simulink model "main_RI_LIEKF"  (R2023a)
settings: Solver=FixedStepAuto  StartTime=0.0  StopTime=220  FixedStep=0.01  RelTol=1e-3
InitFcn:
  | initNavigation0612_AOA;
values from neighbouring files (symbols this model uses):
  CF_enable = 0    [initNavigation.m]
  dt = 0.01    [initNavigation.m]
  dtDelay = -0.03    [initNavigation.m]
  g0 = 9.795    [initNavigation.m]
  gam0_rad = 0/57.3    (= 0)    [initNavigation.m]
  H_sensor_type = 0    [initNavigation.m]
  KF_enable = 1    [initNavigation.m]
  P0 = diag([1*ones(3,1);0.01*ones(3,1);0.1*ones(3,1);0.001*ones(3,1);0.00001*ones(3,1)])    [initNavigation.m]
  P0_RIEKF = diag([1*ones(3,1);0.01*ones(3,1);0.1*ones(3,1);0.001*ones(3,1);0.00001*ones(3,1);      0.01*ones(3,1);[0;2;2]/57.3;[0.1;0.1;0.1]])^2    [initNavigation.m]
  pd0 = 0    [initNavigation.m]
  pe0 = 0    [initNavigation.m]
  phi0_rad = 0/57.3    (= 0)    [initNavigation.m]
  pn0 = 0    [initNavigation.m]
  psi = -178    [initNavigation.m]
  psi0_rad = 0/57.3    (= 0)    [initNavigation.m]
  state_dim = 24    [initNavigation.m]
  Time = 0:0.01:(size(traindata.AttackAngle,1) - 1)*0.01    [NNLiftCoefficientFit.m]
  vd0 = 0    [initNavigation.m]
  ve0 = 0    [initNavigation.m]
  vn0 = 0    [initNavigation.m]
undefined symbols (not defined in the file or in its folder): DiscIntNeverNeededParam, Discrete, INS_CONST, INS_EXPORT, INS_PARAM, magnitude, p, param, pInitialization, sys
libraries: simulink x69, simulink_extras x64, dspstat3 x56, sharedtransform x49, ctrlSharedLib x36, sharedTrackingLibrary x17, FMT_Model_Lib x13, matrix_library x12, deeplib x4, dspsolvers x4, vrlib x4, aerolibconvert2 x1
(part 11 of 22)

== system main_RI_LIEKF/State estimation/RI UKF/INS propogation/att update ==
  dtheta : Inport
  gyro : Inport  Port=2
  quat_0 : Inport  Port=3  PortDimensions=4
  init_flag : Inport  Port=4
  Bus Creator1 : BusCreator  Inputs=1
  Constant : Constant  Value=dt
  Delay1 : Delay  DelayLength=1  InitialConditionSource=Input port  InitialCondition=0  ExternalReset=Level hold
      settings: InputPortMap=u0,r5,p4
  Detect Increase : simulink/Logic and Bit Operations/Detect Increase  vinit=0.0  OutDataTypeStr=boolean
  Gain1 : Gain  Commented=on  Gain=0.1
  MATLAB Function : MATLAB Function  TreatAsAtomicUnit=on
  MATLAB Function2 : MATLAB Function  TreatAsAtomicUnit=on
  Quaternions to Direction Cosine Matrix : sharedtransform/Quaternions to  Direction Cosine Matrix  aMode=aMode
      settings: LibrarySourceBlock=|
      | aerolibtransform2/Quaternions to
      | Direction Cosine Matrix
  Scope : Scope
  Transpose : Math  Operator=transpose
  att_update1 : Outport
  wires:
  init_flag/1 -> Detect Increase/1
  quat_0/1 -> Quaternions to Direction Cosine Matrix/1
  gyro/1 -> MATLAB Function/2(w)  "w"
  Constant/1 -> MATLAB Function/3(dt)
  Quaternions to Direction Cosine Matrix/1 -> Transpose/1
  Transpose/1 -> Delay1/3
  Delay1/1 -> MATLAB Function/1(Rbn_k_1)
  Detect Increase/1 -> Delay1/2
  Bus Creator1/1 -> att_update1/1
  MATLAB Function/1(Rbn) -> MATLAB Function2/2(Rbn)  "DCM_b_n"
  MATLAB Function2/1(Rbn_correct) -> Bus Creator1/1, Delay1/1  "DCM_b_n"
  dtheta/1 -> MATLAB Function2/1(delta), Scope/1

== system main_RI_LIEKF/State estimation/RI UKF/INS propogation/gyro bias compensation ==
  raw <gyro_B_rad/s_LPF> : Inport
  ddg : Inport  Port=2
  Measuemrnt Enable Flag : Inport  Port=3
  QGC_init : Inport  Port=4
  Add1 : Sum
  Data Type Conversion4 : DataTypeConversion  OutDataTypeStr=single  SaturateOnIntegerOverflow=off  RndMeth=Floor
  Scope1 : Scope
  error compensation : Subsystem
      settings: PortSchema="{\"entries\":[{\"content\":{\"sides\":[{\"content\":{\"connectorIds\":[\"In1\",\"In2\"]},\"type\":\"ConnectorPlacement.EquallySpacedRectSide\",\"uuid\":\"380e61a1-8124-48da-8c16-e78a4b6c30a9\"},{\"content\":{\"connectorIds\":[\"Out1\"],\"side\":\"RIGHT\"},\"type\":\"ConnectorPlacement.EquallySpacedRectSide\",\"uuid\":\"dacfd24e-67c3-4852-b5f7-795187362148\"},{\"content\":{\"side\":\"TOP\"},\"type\":\"ConnectorPlacement.EquallySpacedRectSide\",\"uuid\":\"56579dc4-3963-4476-a5d7-e0c30cfcd11c\"},{\"content\":{\"connectorIds\":[\"In3\"],\"side\":\"BOTTOM\"},\"type\":\"ConnectorPlacement.EquallySpacedRectSide\",\"uuid\":\"fc24e139-e918-40f2-99cc-0ca16c0a4a58\"}]},\"type\":\"ConnectorPlacement.EquallySpacedConnector\",\"uuid\":\"3ce5c04a-f8d2-476b-8ef1-0541292dfd95\"}],\"packageUris\":[\"http://schema.mathworks.com/mf0/Connector/R2020b\"],\"version\":\"1.0\"}"
  wb : Outport
  dg : Outport  Port=2
  wires:
  Data Type Conversion4/1 -> wb/1
  raw <gyro_B_rad/s_LPF>/1 -> Add1/1
  error compensation/1(dg) -> Add1/2, Scope1/1, dg/1
  Measuemrnt Enable Flag/1 -> error compensation/2(Enable)
  Add1/1 -> Data Type Conversion4/1
  QGC_init/1 -> error compensation/3(QGC_init)
  ddg/1 -> error compensation/1(ddg)

== system main_RI_LIEKF/State estimation/RI UKF/INS propogation/vel//pos update ==
  dtheta : Inport
  <DCM_b_n> : Inport  Port=2
  Ab : Inport  Port=3
  v0 : Inport  Port=4
  p0 : Inport  Port=5
  QGC_init : Inport  Port=6
  dp : Inport  Port=7
  dv : Inport  Port=8
  Kinematic Equation : Subsystem
  QGC_init1 : InportShadow  Port=6
  pos update : Subsystem
  vel update : Subsystem
  p_k : Outport
  V : Outport  Port=2
  wires:
  QGC_init1/1 -> pos update/4(QGC_init)
  pos update/1(p_k) -> p_k/1
  p0/1 -> pos update/5(p0)
  dp/1 -> pos update/3(dp)
  v0/1 -> vel update/5(v0)
  dv/1 -> vel update/4(KFState_dv)
  Kinematic Equation/1(An) -> vel update/3(An)
  QGC_init/1 -> vel update/2(QGC_init)
  Ab/1 -> Kinematic Equation/2(Ab)
  <DCM_b_n>/1 -> Kinematic Equation/1(Cbn)
  vel update/1(vel_k) -> pos update/2(vel_k), V/1
  dtheta/1 -> pos update/1(dtheta), vel update/1(dtheta)

== system main_RI_LIEKF/State estimation/bak1/Error State Kalman Filter/Cal Q1 ==
  Constant : Constant  Value=dt  OutDataTypeStr=double
  MATLAB Function1 : MATLAB Function  TreatAsAtomicUnit=on
  Qd : Outport
  wires:
  MATLAB Function1/1(Q) -> Qd/1
  Constant/1 -> MATLAB Function1/1(dt)

== system main_RI_LIEKF/State estimation/bak1/Error State Kalman Filter/Extended Kalman Filter1 ==
  Q : Inport
  Enable1 : Inport  Port=2
  y1 : Inport  Port=3
  R1 : Inport  Port=4
  BlockOrdering : Constant  Value=true()  OutDataTypeStr=boolean
  Correct1 : Subsystem  AncestorBlock=sharedTrackingLibrary/Extras/EKFCorrect  TreatAsAtomicUnit=on  SystemSampleTime=p.SampleTimes.MeasurementFcn(1)  mask(EKFCorrect){ProcessedMaskData=p}
      mask init: same as main_RI_LIEKF/State estimation/0609bk/Error State Kalman Filter/Extended Kalman Filter1/Correct1
      settings: LibrarySourceBlock=sharedTrackingLibrary/Extras/EKFCorrect
  DataStoreMemory - P : DataStoreMemory  DataStoreName=P  InitialValue=p.InitialCovariance  ShowAdditionalParam=off  OutDataTypeStr=p.DataType
  DataStoreMemory - x : DataStoreMemory  DataStoreName=x  InitialValue=p.InitialState  ShowAdditionalParam=off  OutDataTypeStr=p.DataType
  DataTypeConversion_Enable1 : DataTypeConversion  OutDataTypeStr=boolean  SaturateOnIntegerOverflow=off  RndMeth=Floor
  DataTypeConversion_Q : DataTypeConversion  OutDataTypeStr=p.DataType  SaturateOnIntegerOverflow=off  RndMeth=Floor
  DataTypeConversion_R1 : DataTypeConversion  OutDataTypeStr=p.DataType  SaturateOnIntegerOverflow=off  RndMeth=Floor
  DataTypeConversion_uMeas1 : DataTypeConversion  OutDataTypeStr=p.DataType  SaturateOnIntegerOverflow=off  RndMeth=Floor
  DataTypeConversion_uState : DataTypeConversion  OutDataTypeStr=p.DataType  SaturateOnIntegerOverflow=off  RndMeth=Floor
  DataTypeConversion_y1 : DataTypeConversion  OutDataTypeStr=p.DataType  SaturateOnIntegerOverflow=off  RndMeth=Floor
  MeasurementFcn1Inputs : Constant  Value=0  OutDataTypeStr=p.DataType  SampleTime=p.SampleTimes.MeasurementFcn(1)
  Output : Subsystem  TreatAsAtomicUnit=on  SystemSampleTime=p.SampleTimes.Output
  Predict : Subsystem  TreatAsAtomicUnit=on  SystemSampleTime=p.SampleTimes.StateTransitionFcn  mask(EKFPredict){ProcessedMaskData=p}
      mask init: same as main_RI_LIEKF/State estimation/0609bk/Error State Kalman Filter/Extended Kalman Filter1/Predict
  StateTransitionFcnInputs : Constant  Value=0  OutDataTypeStr=p.DataType  SampleTime=p.SampleTimes.StateTransitionFcn
  checkMeasurementFcn1Signals : S-Function  FunctionName=ekfukfCheckSignals  Parameters=signalCheck.BlockPath, signalCheck.MeasurementFcn{1}.PortNames, signalCheck.MeasurementFcn{1}.SampleTime, signalCheck.DataType, signalCheck.MeasurementFcn{1}.PortDimensions, 1, signalCheck.MeasurementFcn{1}.HasAdditiveNoise  SFunctionDeploymentMode=off  EnableBusSupport=off
  checkStateTransitionFcnSignals : S-Function  FunctionName=ekfukfCheckSignals  Parameters=signalCheck.BlockPath, signalCheck.StateTransitionFcn.PortNames, signalCheck.StateTransitionFcn.SampleTime, signalCheck.DataType, signalCheck.StateTransitionFcn.PortDimensions, 0, signalCheck.StateTransitionFcn.HasAdditiveNoise  SFunctionDeploymentMode=off  EnableBusSupport=off
  xhat : Outport  VectorParamsAs1DForOutWhenUnconnected=off
  P : Outport  Port=2
  wires:
  Correct1/1(yBlockOrdering) -> [AfterCorrect]
  y1/1 -> checkMeasurementFcn1Signals/2, DataTypeConversion_y1/1
  R1/1 -> checkMeasurementFcn1Signals/3, DataTypeConversion_R1/1
  Q/1 -> checkStateTransitionFcnSignals/1, DataTypeConversion_Q/1
  DataTypeConversion_Q/1 -> Predict/1(Q)
  Enable1/1 -> checkMeasurementFcn1Signals/1, DataTypeConversion_Enable1/1
  DataTypeConversion_Enable1/1 -> Correct1/Enable
  Output/2(P) -> P/1
  Output/1(x) -> xhat/1
  StateTransitionFcnInputs/1 -> checkStateTransitionFcnSignals/2, DataTypeConversion_uState/1
  DataTypeConversion_uState/1 -> Predict/2(uState)
  DataTypeConversion_y1/1 -> Correct1/1(yMeas)
  MeasurementFcn1Inputs/1 -> checkMeasurementFcn1Signals/4, DataTypeConversion_uMeas1/1
  DataTypeConversion_R1/1 -> Correct1/2(R)
  DataTypeConversion_uMeas1/1 -> Correct1/3(uMeas)
  BlockOrdering/1 -> [FirstOperation]
  [FirstOperation] -> Correct1/4(uBlockOrdering)
  [AfterCorrect] -> Output/1(uBlockOrdering)
  Output/3(yBlockOrdering) -> [AfterOutput]
  [AfterOutput] -> Predict/3(uBlockOrdering)

== system main_RI_LIEKF/State estimation/bak1/Error State Kalman Filter/Simulink Function - GPS Measurements ==
  Rbn : Inport
  vn : Inport  Port=2
  pn : Inport  Port=3
  GPSMeasurementFcn_Dyn : TriggerPort  TriggerType=function-call  IsSimulinkFunction=on  FunctionName=GPSMeasurementFcn_Dyn  VariantControl=Variant
  Add : Sum
  Data Type Conversion1 : DataTypeConversion  OutDataTypeStr=single  SaturateOnIntegerOverflow=off  RndMeth=Floor
  MATLAB Function : MATLAB Function  TreatAsAtomicUnit=on
  MATLAB Function1 : MATLAB Function  Commented=on  TreatAsAtomicUnit=on
  Product : Product  Multiplication=Matrix(*)
  pn1 : InportShadow  Port=3
  vn1 : InportShadow  Port=2
  x : ArgIn  DisableCoverage=on  OutDataTypeStr=single  PortDimensions=15  ArgumentName=x
  v : ArgIn  DisableCoverage=on  Port=2  OutDataTypeStr=single  PortDimensions=6  ArgumentName=v
  y : ArgOut  DisableCoverage=on  OutDataTypeStr=single  PortDimensions=6  ArgumentName=y
  wires:
  Data Type Conversion1/1 -> Product/1
  pn/1 -> MATLAB Function/2(pn)
  v/1 -> Add/2
  x/1 -> Product/2
  pn1/1 -> MATLAB Function1/3(pn)
  vn1/1 -> MATLAB Function1/2(vn)
  Rbn/1 -> MATLAB Function1/1(Rbn)
  vn/1 -> MATLAB Function/1(vn)
  Add/1 -> y/1
  Product/1 -> Add/1
  MATLAB Function/1(H) -> Data Type Conversion1/1

== system main_RI_LIEKF/State estimation/bak1/Error State Kalman Filter/Simulink Function - GPS Measurements1 ==
  DCM_b_n : Inport
  DynamicMeasurementFcn_Dyn : TriggerPort  TriggerType=function-call  IsSimulinkFunction=on  FunctionName=DynamicMeasurementFcn_Dyn  VariantControl=Variant
  Add : Sum  Commented=on
  Add1 : Sum
  Constant : Constant  Commented=on  Value=dt  OutDataTypeStr=single
  Constant6 : Constant  Value=[zeros(3,3),eye(3),zeros(3,12);zeros(3,15),eye(3)]  OutDataTypeStr=single
  Data Type Conversion6 : DataTypeConversion  Commented=on  OutDataTypeStr=single  SaturateOnIntegerOverflow=off  RndMeth=Floor
  From7 : From  Commented=on  GotoTag=DCM_b_n
  Goto : Goto  Commented=on  GotoTag=DCM_b_n
  MATLAB Function1 : MATLAB Function  Commented=on  TreatAsAtomicUnit=on
  Product : Product  Commented=on  Multiplication=Matrix(*)
  Product1 : Product  Multiplication=Matrix(*)
  x : ArgIn  DisableCoverage=on  OutDataTypeStr=single  PortDimensions=18  ArgumentName=x
  v : ArgIn  DisableCoverage=on  Port=2  OutDataTypeStr=single  PortDimensions=6  ArgumentName=v
  y : ArgOut  DisableCoverage=on  OutDataTypeStr=single  PortDimensions=6  ArgumentName=y
  wires:
  x/1 -> Product1/2
  Constant6/1 -> Product1/1
  Product1/1 -> Add1/1
  v/1 -> Add1/2
  Add1/1 -> y/1
  Data Type Conversion6/1 -> Product/1
  DCM_b_n/1 -> Goto/1
  Constant/1 -> MATLAB Function1/2(dt)
  From7/1 -> MATLAB Function1/1(Cbn)
  MATLAB Function1/1(H) -> Data Type Conversion6/1
  Product/1 -> Add/1

== system main_RI_LIEKF/State estimation/bak1/Error State Kalman Filter/Simulink Function - GPS Measurements2 ==
  ZUPTMeasurementFcn2 : TriggerPort  TriggerType=function-call  IsSimulinkFunction=on  FunctionName=ZUPTMeasurementFcn2  VariantControl=Variant
  Add : Sum
  Constant6 : Constant  Value=[zeros(3,3),eye(3),zeros(3,12)]  OutDataTypeStr=single
  Product : Product  Multiplication=Matrix(*)
  x : ArgIn  DisableCoverage=on  OutDataTypeStr=single  PortDimensions=18  ArgumentName=x
  v : ArgIn  DisableCoverage=on  Port=2  OutDataTypeStr=single  PortDimensions=3  ArgumentName=v
  y : ArgOut  DisableCoverage=on  OutDataTypeStr=single  PortDimensions=3  ArgumentName=y
  wires:
  v/1 -> Add/2
  Constant6/1 -> Product/1
  x/1 -> Product/2
  Product/1 -> Add/1
  Add/1 -> y/1

== system main_RI_LIEKF/State estimation/bak1/Error State Kalman Filter/Simulink Function - State Transition ==
  DCM_b_n : Inport
  vn : Inport  Port=2  PortDimensions=[3,1]
  pn : Inport  Port=3  PortDimensions=[3,1]
  stateTransitionFcn_Dyn : TriggerPort  TriggerType=function-call  IsSimulinkFunction=on  FunctionName=stateTransitionFcn_Dyn  VariantControl=Variant
  Add : Sum
  Cal Phi : Subsystem
  Constant : Constant  Value=dt  OutDataTypeStr=single
  Data Type Conversion1 : DataTypeConversion  OutDataTypeStr=single  SaturateOnIntegerOverflow=off  RndMeth=Floor
  Data Type Conversion6 : DataTypeConversion  OutDataTypeStr=single  SaturateOnIntegerOverflow=off  RndMeth=Floor
  MATLAB Function : MATLAB Function  TreatAsAtomicUnit=on
  Product1 : Product  Multiplication=Matrix(*)
  Product2 : Product  Multiplication=Matrix(*)
  x : ArgIn  DisableCoverage=on  OutDataTypeStr=single  PortDimensions=15  ArgumentName=x
  w : ArgIn  Port=2  OutDataTypeStr=single  PortDimensions=12  ArgumentName=w
  xNext : ArgOut  DisableCoverage=on  OutDataTypeStr=single  PortDimensions=15  ArgumentName=xNext
  wires:
  pn/1 -> Cal Phi/3(pn), MATLAB Function/3(pn)
  vn/1 -> Cal Phi/2(vn), MATLAB Function/2(vn)
  [DCM_b_n] -> Cal Phi/1(Rbn)
  Data Type Conversion6/1 -> Add/2
  Data Type Conversion1/1 -> Add/1
  Cal Phi/1(Phi) -> Product2/1
  DCM_b_n/1 -> [DCM_b_n]
  Constant/1 -> MATLAB Function/4(dt)
  [DCM_b_n] -> MATLAB Function/1(Rbn)
  Add/1 -> xNext/1
  Product1/1 -> Data Type Conversion1/1
  w/1 -> Product1/2
  MATLAB Function/1(G) -> Product1/1
  Product2/1 -> Data Type Conversion6/1
  x/1 -> Product2/2

== system main_RI_LIEKF/State estimation/bak1/Error State Kalman Filter/Simulink Function - State Transition Jacobian ==
  DCM_b_n : Inport
  wxyz : Inport  Port=2
  fbxyz : Inport  Port=3
  stateTransitionJacobianFcn_Dyn : TriggerPort  TriggerType=function-call  IsSimulinkFunction=on  FunctionName=stateTransitionJacobianFcn_Dyn  VariantControl=Variant
  Cal Phi : Subsystem
  Constant : Constant  Value=0.01  OutDataTypeStr=single
  Data Type Conversion1 : DataTypeConversion  OutDataTypeStr=single  SaturateOnIntegerOverflow=off  RndMeth=Floor
  Data Type Conversion6 : DataTypeConversion  OutDataTypeStr=single  SaturateOnIntegerOverflow=off  RndMeth=Floor
  MATLAB Function : MATLAB Function  TreatAsAtomicUnit=on
  Terminator : Terminator
  Terminator1 : Terminator
  Transpose : Math  Operator=transpose
  x : ArgIn  DisableCoverage=on  OutDataTypeStr=single  PortDimensions=18  ArgumentName=x
  w : ArgIn  Port=2  OutDataTypeStr=single  PortDimensions=15  ArgumentName=w
  A : ArgOut  DisableCoverage=on  OutDataTypeStr=single  PortDimensions=[18 18]  ArgumentName=A
  G : ArgOut  Port=2  OutDataTypeStr=single  PortDimensions=[18 15]  ArgumentName=G
  wires:
  Data Type Conversion1/1 -> G/1
  Data Type Conversion6/1 -> A/1
  Constant/1 -> MATLAB Function/3(dt)
  Transpose/1 -> MATLAB Function/1(Cnb)
  [DCM_b_n] -> Transpose/1
  [wxyz] -> MATLAB Function/2(wxyz)
  [DCM_b_n] -> Cal Phi/1(<DCM_b_n>)
  [fbxyz] -> Cal Phi/3(axyz)
  [wxyz] -> Cal Phi/2(wxyz)
  wxyz/1 -> [wxyz]
  fbxyz/1 -> [fbxyz]
  DCM_b_n/1 -> [DCM_b_n]
  Cal Phi/1(Phi) -> Data Type Conversion6/1
  w/1 -> Terminator1/1
  x/1 -> Terminator/1
  MATLAB Function/1(G) -> Data Type Conversion1/1

== system main_RI_LIEKF/State estimation/bak1/Error State Kalman Filter/Subsystem ==
  data : Inport
  Detect Change : simulink/Logic and Bit Operations/Detect Change  vinit=0  InputProcessing=Columns as channels (frame based)  OutDataTypeStr=boolean
  Selector : Selector  InputPortWidth=3  IndexOptions=Index vector (dialog)  Indices=[3]  OutputSizes=1
  Zero-Order Hold : ZeroOrderHold  SampleTime=0.2
  Zero-Order Hold1 : ZeroOrderHold  SampleTime=0.01
  flag : Outport
  wires:
  Zero-Order Hold/1 -> Selector/1
  data/1 -> Zero-Order Hold/1
  Selector/1 -> Zero-Order Hold1/1
  Detect Change/1 -> flag/1
  Zero-Order Hold1/1 -> Detect Change/1

== system main_RI_LIEKF/State estimation/bak1/INS propogation/Init_PVQ ==
  QGC_sensor_reinit : Inport
  accl_B_m/s2_LPF : Inport  Port=2
  Magn_B_guess_LPF : Inport  Port=3
  pos_NED : Inport  Port=4
  vel_NED : Inport  Port=5
  Constant : Constant  Value=[1 0 0 0]  OutDataTypeStr=single
  Constant1 : Constant  OutDataTypeStr=uint8
  Constant2 : Constant  Value=[0;0;0]  OutDataTypeStr=single
  Constant3 : Constant  Value=[0;0;0]  OutDataTypeStr=single
  Detect Increase : simulink/Logic and Bit Operations/Detect Increase  vinit=0.0  OutDataTypeStr=boolean
  Horizontal_attitude : Subsystem  TreatAsAtomicUnit=on
  Memory : Memory
  Scope : Scope  NumInputPorts=2
  Scope1 : Scope
  Scope2 : Scope
  Subsystem : Subsystem
  Subsystem1 : Subsystem
  Switch{,1..3} (4 alike) : Switch  Criteria=u2 > Threshold  SaturateOnIntegerOverflow=off  InputSameDT=off
  quat_0 : Outport
  v0 : Outport  Port=2
  p0 : Outport  Port=3
  wires:
  Subsystem1/1(mean_data) -> Horizontal_attitude/2(Magn_mean_B_guess_LPF)
  Subsystem/1(mean_data) -> Horizontal_attitude/1(accl_mean_B_m/s_LPF)
  Memory/1 -> Switch1/3
  Switch/1 -> quat_0/1, Scope2/1
  Horizontal_attitude/1(quat_0) -> Switch/1
  Constant/1 -> Switch/3
  Constant1/1 -> Switch1/1
  Switch1/1 -> Memory/1, Switch2/2, Switch3/2, Switch/2, Scope1/1
  accl_B_m/s2_LPF/1 -> Subsystem/1(data)
  QGC_sensor_reinit/1 -> Detect Increase/1, Scope/1
  Magn_B_guess_LPF/1 -> Subsystem1/1(data)
  Detect Increase/1 -> Horizontal_attitude/Enable, Switch1/2, Scope/2
  Constant2/1 -> Switch2/3
  Constant3/1 -> Switch3/3
  Switch2/1 -> v0/1
  Switch3/1 -> p0/1
  pos_NED/1 -> Switch3/1
  vel_NED/1 -> Switch2/1

== system main_RI_LIEKF/State estimation/bak1/INS propogation/accl bias compensation ==
  raw <accl_B_m/s2_LPF> : Inport
  dda : Inport  Port=2
  Add2 : Sum
  Data Type Conversion6 : DataTypeConversion  OutDataTypeStr=single  SaturateOnIntegerOverflow=off  RndMeth=Floor
  error compensation1 : Subsystem
  fb : Outport
  da : Outport  Port=2
  wires:
  error compensation1/1(da) -> Add2/2, da/1
  Add2/1 -> Data Type Conversion6/1
  Data Type Conversion6/1 -> fb/1
  raw <accl_B_m/s2_LPF>/1 -> Add2/1
  dda/1 -> error compensation1/1(dda)

== system main_RI_LIEKF/State estimation/bak1/INS propogation/att_update ==
  dtheta : Inport
  gyro : Inport  Port=2
  quat_0 : Inport  Port=3  PortDimensions=4
  init_flag : Inport  Port=4
  Bus Creator1 : BusCreator  Inputs=1
  Constant : Constant  Value=dt
  Delay1 : Delay  DelayLength=1  InitialConditionSource=Input port  InitialCondition=0  ExternalReset=Level hold
      settings: InputPortMap=u0,r5,p4
  Detect Increase : simulink/Logic and Bit Operations/Detect Increase  vinit=0.0  OutDataTypeStr=boolean
  MATLAB Function : MATLAB Function  TreatAsAtomicUnit=on
  MATLAB Function2 : MATLAB Function  TreatAsAtomicUnit=on
  Quaternions to Direction Cosine Matrix : sharedtransform/Quaternions to  Direction Cosine Matrix  aMode=aMode
      settings: LibrarySourceBlock=|
      | aerolibtransform2/Quaternions to
      | Direction Cosine Matrix
  Scope : Scope
  Transpose : Math  Operator=transpose
  att_update1 : Outport
  wires:
  dtheta/1 -> MATLAB Function2/1(delta), Scope/1
  MATLAB Function2/1(Rbn_correct) -> Delay1/1, Bus Creator1/1  "DCM_b_n"
  MATLAB Function/1(Rbn) -> MATLAB Function2/2(Rbn)  "DCM_b_n"
  Bus Creator1/1 -> att_update1/1
  Detect Increase/1 -> Delay1/2
  Delay1/1 -> MATLAB Function/1(Rbn_k_1)
  Transpose/1 -> Delay1/3
  Quaternions to Direction Cosine Matrix/1 -> Transpose/1
  Constant/1 -> MATLAB Function/3(dt)
  gyro/1 -> MATLAB Function/2(w)  "w"
  quat_0/1 -> Quaternions to Direction Cosine Matrix/1
  init_flag/1 -> Detect Increase/1

== system main_RI_LIEKF/State estimation/bak1/INS propogation/gyro bias compensation ==
  raw <gyro_B_rad/s_LPF> : Inport
  ddg : Inport  Port=2
  Measuemrnt Enable Flag : Inport  Port=3
  Add1 : Sum
  Data Type Conversion4 : DataTypeConversion  OutDataTypeStr=single  SaturateOnIntegerOverflow=off  RndMeth=Floor
  Scope1 : Scope
  error compensation : Subsystem
  wb : Outport
  dg : Outport  Port=2
  wires:
  ddg/1 -> error compensation/1(ddg)
  Add1/1 -> Data Type Conversion4/1
  Measuemrnt Enable Flag/1 -> error compensation/2(Enable)
  error compensation/1(dg) -> dg/1, Scope1/1, Add1/2
  raw <gyro_B_rad/s_LPF>/1 -> Add1/1
  Data Type Conversion4/1 -> wb/1

== system main_RI_LIEKF/State estimation/bak1/INS propogation/vel_pos_update ==
  dtheta : Inport
  <DCM_b_n> : Inport  Port=2
  Ab : Inport  Port=3
  v0 : Inport  Port=4
  p0 : Inport  Port=5
  QGC_init : Inport  Port=6
  dp : Inport  Port=7
  dv : Inport  Port=8
  Kinematic Equation : Subsystem
  QGC_init1 : InportShadow  Port=6
  pos update : Subsystem
  vel update : Subsystem
  p_k : Outport
  V : Outport  Port=2
  wires:
  dtheta/1 -> vel update/1(dtheta), pos update/1(dtheta)
  vel update/1(vel_k) -> V/1, pos update/2(vel_k)
  <DCM_b_n>/1 -> Kinematic Equation/1(Cbn)
  Ab/1 -> Kinematic Equation/2(Ab)
  QGC_init/1 -> vel update/2(QGC_init)
  Kinematic Equation/1(An) -> vel update/3(An)
  dv/1 -> vel update/4(KFState_dv)
  v0/1 -> vel update/5(v0)
  dp/1 -> pos update/3(dp)
  p0/1 -> pos update/5(p0)
  pos update/1(p_k) -> p_k/1
  QGC_init1/1 -> pos update/4(QGC_init)

== system main_RI_LIEKF/State estimation/distribute CF/AHRS/AHRS Complementary filter ==
  fbxyz : Inport
  Q_update : Inport  Port=2
  GPS_Data : Inport  Port=3
  magxyz : Inport  Port=4
  reset : Inport  Port=5
  Bus Selector : BusSelector  OutputSignals=vn_gps,ve_gps,vd_gps
  Bus Selector1 : BusSelector  OutputSignals=DCM_b_n
  Bus Selector2 : BusSelector  OutputSignals=fixtype_gps
  Compare To Constant : simulink/Logic and Bit Operations/Compare To Constant  relop=<=  const=2  OutDataTypeStr=boolean
  Complementary Filter : Subsystem
  Constant : Constant  Value=zeros(3,1)  OutDataTypeStr=single
  Discrete-Time Integrator2 : DiscreteIntegrator  Commented=on  ExternalReset=rising  SampleTime=-1  LimitOutput=on  UpperSaturationLimit=0.005  LowerSaturationLimit=-0.005  ICPrevOutput=DiscIntNeverNeededParam  ICPrevScaledInput=DiscIntNeverNeededParam
  GPSHeadingCorrect : Subsystem
  Gain1 : Gain  Gain=[1;1;0]
  Gain3 : Gain  Commented=on  Gain=0.01
  MagnHeadingCorrect : Subsystem
  Q_update1 : InportShadow  Port=2
  Scope{,2..4,6} (5 alike) : Scope
  Scope1 : Scope  NumInputPorts=2
  Scope5 : Scope  NumInputPorts=2
  Sum : Sum  Inputs=|+--
  Switch : Switch  Threshold=3  SaturateOnIntegerOverflow=off  InputSameDT=off
  Terminator1 : Terminator
  Trace differentiator : Subsystem
  UAV_accelerate_within_gravity_estimate : Subsystem
  Vector Concatenate : Concatenate  NumInputs=3
  fbxyz1 : InportShadow
  gyro_preprocessing2 : Subsystem
  manoeuvrable check : Subsystem
  w_bias : Outport
  wires:
  Switch/1 -> Gain1/1
  gyro_preprocessing2/1(gyro_B_rad/s_LPF) -> Gain3/1, w_bias/1, Scope6/1
  Complementary Filter/1(w_bias) -> Switch/3
  reset/1 -> Discrete-Time Integrator2/2
  Constant/1 -> Switch/1
  Sum/1 -> gyro_preprocessing2/1(gyro_B_rad/s_ori)
  Gain3/1 -> Discrete-Time Integrator2/1
  MagnHeadingCorrect/1(wz_bias_by_magn) -> Scope1/1, Sum/3
  magxyz/1 -> MagnHeadingCorrect/2(Magnxyz), Scope1/2
  GPSHeadingCorrect/2(PsiGPS&pitch&roll) -> Terminator1/1
  GPSHeadingCorrect/1(wz_bias_by_GPS) -> Sum/2, Scope/1
  Q_update1/1 -> GPSHeadingCorrect/2(Q_update)
  Gain1/1 -> Sum/1
  manoeuvrable check/1(Fly_status) -> Compare To Constant/1, Switch/2, Scope3/1, Complementary Filter/2(Fly_status), UAV_accelerate_within_gravity_estimate/1(Fly_status)
  Bus Selector2/1 -> manoeuvrable check/4(fixtype_GPS), UAV_accelerate_within_gravity_estimate/2(GPS_type)  "<fixtype_gps>"
  fbxyz1/1 -> manoeuvrable check/2(fbxyz1)
  Trace differentiator/1(originalVariableDifference) -> UAV_accelerate_within_gravity_estimate/4(accel_GPS_ned), manoeuvrable check/1(accel_GPS_ned), Scope5/1  "accel_GPS_ned"
  UAV_accelerate_within_gravity_estimate/1(accelerate_within_gravity_estimate) -> Scope2/1, Complementary Filter/3(fb_estimatedValue)
  fbxyz/1 -> Complementary Filter/1(fbxyz)
  Vector Concatenate/1 -> Trace differentiator/1(originalVariable), Scope5/2, Scope4/1  "v_GPS_ned"
  Bus Selector1/1 -> MagnHeadingCorrect/1(Cbn), manoeuvrable check/3(DCM_b_n), UAV_accelerate_within_gravity_estimate/3(<DCM_b_n>)  "<DCM_b_n>"
  Q_update/1 -> Bus Selector1/1
  Bus Selector/3 -> Vector Concatenate/3  "<vd_gps>"
  Bus Selector/2 -> Vector Concatenate/2  "<ve_gps>"
  Bus Selector/1 -> Vector Concatenate/1  "<vn_gps>"
  GPS_Data/1 -> Bus Selector/1, GPSHeadingCorrect/1(GPSdata), Bus Selector2/1

== system main_RI_LIEKF/State estimation/distribute CF/AHRS/Init_Q0 ==
  QGC_sensor_reinit : Inport
  accl_B_m/s2_LPF : Inport  Port=2
  Magn_B_guess_LPF : Inport  Port=3
  Constant : Constant  Value=[1 0 0 0]  OutDataTypeStr=single
  Constant1 : Constant  OutDataTypeStr=uint8
  Detect Increase : simulink/Logic and Bit Operations/Detect Increase  vinit=0.0  OutDataTypeStr=boolean
  Horizontal_attitude : Subsystem  TreatAsAtomicUnit=on
  Memory : Memory
  Scope : Scope  NumInputPorts=2
  Scope1 : Scope
  Scope2 : Scope
  Subsystem : Subsystem
  Subsystem1 : Subsystem
  Switch : Switch  Criteria=u2 > Threshold  SaturateOnIntegerOverflow=off  InputSameDT=off
  Switch1 : Switch  Criteria=u2 > Threshold  SaturateOnIntegerOverflow=off  InputSameDT=off
  quat_0 : Outport
  wires:
  Subsystem1/1(mean_data) -> Horizontal_attitude/2(Magn_mean_B_guess_LPF)
  Subsystem/1(mean_data) -> Horizontal_attitude/1(accl_mean_B_m/s_LPF)
  Memory/1 -> Switch1/3
  Switch/1 -> quat_0/1, Scope2/1
  Horizontal_attitude/1(quat_0) -> Switch/1
  Constant/1 -> Switch/3
  Constant1/1 -> Switch1/1
  Switch1/1 -> Memory/1, Switch/2, Scope1/1
  accl_B_m/s2_LPF/1 -> Subsystem/1(data)
  QGC_sensor_reinit/1 -> Detect Increase/1, Scope/1
  Magn_B_guess_LPF/1 -> Subsystem1/1(data)
  Detect Increase/1 -> Horizontal_attitude/Enable, Switch1/2, Scope/2

== system main_RI_LIEKF/State estimation/distribute CF/AHRS/att_update ==
  Sensor_data : Inport
  quat_0 : Inport  Port=2  PortDimensions=4
  init_flag : Inport  Port=3
  wbias : Inport  Port=4  PortDimensions=3
  Add : Sum
  Bus Creator : BusCreator  Inputs=2
  Bus Selector1 : BusSelector  OutputSignals=IMU_Data.gyro_B_rad/s_LPF
  Delay : Delay  DelayLength=1  InitialConditionSource=Input port  ExternalReset=Level hold
      settings: InputPortMap=u0,r5,p4
  Detect Increase : simulink/Logic and Bit Operations/Detect Increase  vinit=0.0  OutDataTypeStr=boolean
  Gain : Gain  Gain=dt
  Memory : Memory  InitialCondition=zeros(3,1)  InheritSampleTime=on
  QuatMult : MATLAB Function  TreatAsAtomicUnit=on
  Quaternions to Direction Cosine Matrix : sharedtransform/Quaternions to  Direction Cosine Matrix  aMode=aMode
  Scope : Scope
  Scope1 : Scope
  Transpose : Math  Operator=transpose  SignedPower=on
  rv2q : MATLAB Function  TreatAsAtomicUnit=on
  uniformization : Subsystem
  att_update : Outport
  wires:
  uniformization/1(Q o) -> Bus Creator/1, Delay/1, Quaternions to Direction Cosine Matrix/1  "q_update"
  Memory/1 -> Add/2
  wbias/1 -> Memory/1
  Detect Increase/1 -> Delay/2
  init_flag/1 -> Detect Increase/1
  Bus Creator/1 -> att_update/1
  Transpose/1 -> Bus Creator/2  "DCM_b_n"
  Quaternions to Direction Cosine Matrix/1 -> Transpose/1
  quat_0/1 -> Delay/3
  Delay/1 -> QuatMult/1(quatA)
  QuatMult/1(quatOut) -> uniformization/1(Q i)  "q_update"
  Sensor_data/1 -> Bus Selector1/1
  Gain/1 -> rv2q/1(rotVec)  "correctedDelAng"
  Bus Selector1/1 -> Add/1, Scope1/1  "<gyro_B_rad/s_LPF>"
  Add/1 -> Gain/1
  rv2q/1(quaternion) -> QuatMult/2(quatB)

== system main_RI_LIEKF/State estimation/distribute CF/Translation_estimate/Rxy_Horizontal_estimation ==
  Vn : Inport
  Enable : Inport  Port=2
  Sensor_data2 : Inport  Port=3
  Add1 : Sum  Inputs=+-
  Bus Selector1 : BusSelector  OutputSignals=GPS_Data.pos_N_gps,GPS_Data.pos_E_gps
  Delay1 : Delay  DelayLength=1
  Integrator_R_Horizontal : Subsystem
  Mux1 : Mux  Inputs=2
  Rxy_kalman filter2 : Subsystem  mask{F=diag([-0.1,-0.1,-0.01,-0.01]), H=[1,0,-1,0;0,1,0,-1], Q=diag([1,1,0.1,0.1]), R=diag([0.05,0.05]), P0=diag([0.8,0.8,0.2,0.2])}
      mask prompts: F "状态转移矩阵：F"; H "观测转移矩阵：H"; Q "预测噪声协方差矩阵：Q"; R "量测噪声协方差矩阵：R"; P0 "初始协方差矩阵：P0"
      mask DialogControl DescTextVar Prompt: Kalman Filter
  Scope1 : Scope  NumInputPorts=2
  Selector1 : Selector  InputPortWidth=4  IndexOptions=Index vector (dialog)  Indices=[1 2]  OutputSizes=1
  R_n&e : Outport
  wires:
  Vn/1 -> Integrator_R_Horizontal/1(Vn)
  Add1/1 -> Rxy_kalman filter2/2(Z)
  Rxy_kalman filter2/1(XOut) -> Delay1/1
  Enable/1 -> Rxy_kalman filter2/3(Enable)
  Bus Selector1/1 -> Mux1/1  "<pos_N_gps>"
  Integrator_R_Horizontal/1(R_n&e) -> Add1/1, Scope1/1, R_n&e/1
  Bus Selector1/2 -> Mux1/2  "<pos_E_gps>"
  Sensor_data2/1 -> Bus Selector1/1, Integrator_R_Horizontal/3(Sensor_data2)
  Delay1/1 -> Rxy_kalman filter2/1(X), Selector1/1
  Mux1/1 -> Scope1/2, Add1/2
  Selector1/1 -> Integrator_R_Horizontal/2(dR)

== system main_RI_LIEKF/State estimation/distribute CF/Translation_estimate/V_Horizontal_estimation ==
  note: 0530改：
      | 加入GPStype限制
  An : Inport
  Sensor_data2 : Inport  Port=2
  Add : Sum  Inputs=+-
  Bus Selector2 : BusSelector  OutputSignals=GPS_Data.vn_gps,GPS_Data.ve_gps,GPS_Data.fixtype_gps
  Compare To Constant : simulink/Logic and Bit Operations/Compare To Constant  relop=>=  const=1  OutDataTypeStr=boolean
  Delay : Delay  DelayLength=1
  Detect Change : simulink/Logic and Bit Operations/Detect Change  vinit=0  OutDataTypeStr=boolean
  Integrator_V_Horizontal : Subsystem
  Logical Operator : Logic  AllPortsSameDT=off  OutDataTypeStr=boolean
  Mux : Mux  Inputs=2
  Rxy_kalman filter1 : Subsystem  mask{F=diag([-0.1,-0.1,-0.01,-0.01]), H=[1,0,-1,0;0,1,0,-1], Q=diag([1,1,0.1,0.1]), R=diag([0.1,0.1]), P0=diag([0.8,0.8,0.5,0.5])}
      mask prompts: F "状态转移矩阵：F"; H "观测转移矩阵：H"; Q "预测噪声协方差矩阵：Q"; R "量测噪声协方差矩阵：R"; P0 "初始协方差矩阵：P0"
      mask DialogControl DescTextVar Prompt: Kalman Filter
  Scope : Scope  NumInputPorts=2
  Scope1 : Scope
  Selector : Selector  InputPortWidth=4  IndexOptions=Index vector (dialog)  Indices=[1 2]  OutputSizes=1
  vxy_estimout : Outport
  V_n&e : Outport  Port=2
  GPS_v_enable : Outport  Port=3
  wires:
  Logical Operator/1 -> Rxy_kalman filter1/3(Enable), Scope1/1, GPS_v_enable/1
  Compare To Constant/1 -> Logical Operator/2
  Detect Change/1 -> Logical Operator/1
  Bus Selector2/3 -> Compare To Constant/1  "<fixtype_gps>"
  Sensor_data2/1 -> Integrator_V_Horizontal/3(Sensor_data2), Bus Selector2/1
  An/1 -> Integrator_V_Horizontal/1(An)
  Add/1 -> Rxy_kalman filter1/2(Z)
  Integrator_V_Horizontal/1(V_n&e) -> Add/1, Scope/1, vxy_estimout/1, V_n&e/1
  Rxy_kalman filter1/1(XOut) -> Delay/1
  Bus Selector2/2 -> Mux/2  "<ve_gps>"
  Mux/1 -> Add/2, Scope/2
  Bus Selector2/1 -> Detect Change/1, Mux/1  "<vn_gps>"
  Selector/1 -> Integrator_V_Horizontal/2(dv)
  Delay/1 -> Rxy_kalman filter1/1(X), Selector/1

== system main_RI_LIEKF/State estimation/distribute CF/Translation_estimate/translate to N ==
  RotationData : Inport
  Sensor_data : Inport  Port=2
  Bus Selector2 : BusSelector  OutputSignals=IMU_Data.accl_B_m/s2_LPF
  Bus Selector3 : BusSelector  OutputSignals=DCM_b_n
  Product : Product  Multiplication=Matrix(*)
  Selector : Selector  InputPortWidth=3  IndexOptions=Index vector (dialog)  Indices=[1 2]  OutputSizes=1
  Selector1 : Selector  InputPortWidth=3  IndexOptions=Index vector (dialog)  Indices=[3]  OutputSizes=1
  accel_Horizontal_predict : Outport
  accel_Vertical_predict : Outport  Port=2
  wires:
  Selector1/1 -> accel_Vertical_predict/1
  Selector/1 -> accel_Horizontal_predict/1
  Product/1 -> Selector/1, Selector1/1
  Sensor_data/1 -> Bus Selector2/1
  Bus Selector3/1 -> Product/1  "<DCM_b_n>"
  Bus Selector2/1 -> Product/2  "<accl_B_m/s2_LPF>"
  RotationData/1 -> Bus Selector3/1

== system main_RI_LIEKF/State estimation/distribute CF/distribute CF/AHRS1 ==
  RF_Data : Inport
  Sensor_Data : Inport  Port=2
  Bus_Constructor : Subsystem  TreatAsAtomicUnit=on
  Correct : Subsystem  TreatAsAtomicUnit=on
  Delay : Delay  DelayLength=1
  Update : Subsystem  TreatAsAtomicUnit=on
  Rotation_Data : Outport
  wires:
  Correct/1(att_B_correction) -> Update/1(att_B_correction)
  Bus_Constructor/1(Rotation_Data) -> Delay/1, Rotation_Data/1
  Correct/2(bias_g_B_correction) -> Update/2(bias_g_correction)
  Sensor_Data/1 -> Bus_Constructor/5(Sensor_Data), Update/4(Sensor_Data), Correct/2(Sensor_Data)
  Update/1(att_quat) -> Bus_Constructor/2(att_quat)
  Update/2(DCM_OB) -> Bus_Constructor/3(DCM_OB)
  Update/3(bias_g) -> Bus_Constructor/4(bias_g)
  RF_Data/1 -> Correct/3(RF_Data), Bus_Constructor/1(RF_Data), Update/3(RF_Data)
  Delay/1 -> Correct/1(Rotation_Data)

== system main_RI_LIEKF/State estimation/distribute CF/distribute CF/Bus_Constructor ==
  RF_Data : Inport
  att_quat : Inport  Port=2
  DCM_OB : Inport  Port=3
  bias_g : Inport  Port=4
  gyro_B_correction : Inport  Port=5
  Sensor_Data : Inport  Port=6
  Bus Creator : BusCreator  Inputs=12
  Bus Selector : BusSelector  OutputSignals=IMU_Data.gyro_B_rad/s_LPF,IMU_Data.accl_B_m/s2_LPF
  Bus Selector1 : BusSelector  OutputSignals=att_reset
  Constant : Constant
  Euler_Angle : Subsystem
  Math Function : Math  Operator=transpose  SignedPower=on
  Signal Conversion{,1..4} (5 alike) : SignalConversion  OverrideOpt=off
  Subsystem1 : Subsystem
  Terminator2 : Terminator
  Rotation_Data : Outport
  wires:
  Bus Selector1/1 -> Signal Conversion4/1  "<att_reset>"
  Signal Conversion/1 -> Bus Creator/11  "acc_B_mPs2"
  Euler_Angle/1(phi_rad) -> Bus Creator/2  "phi_rad"
  Euler_Angle/2(theta_rad) -> Bus Creator/3  "theta_rad"
  Euler_Angle/3(psi_rad) -> Subsystem1/1(psi), Bus Creator/4  "psi_rad"
  Sensor_Data/1 -> Bus Selector/1
  Bus Creator/1 -> Rotation_Data/1
  bias_g/1 -> Signal Conversion3/1
  Math Function/1 -> Bus Creator/7  "M_BO"
  DCM_OB/1 -> Math Function/1, Bus Creator/8  "M_OB"
  att_quat/1 -> Euler_Angle/1(att_quat), Bus Creator/6  "att_quat"
  Subsystem1/1(DCMz) -> Bus Creator/5  "M_CO"
  Signal Conversion1/1 -> Bus Creator/12  "standstill"
  Bus Selector/2 -> Signal Conversion/1  "<accl_B_m/s2_LPF>"
  Signal Conversion2/1 -> Bus Creator/10  "gyr_B_radPs"
  Signal Conversion3/1 -> Bus Creator/9  "bias_g"
  RF_Data/1 -> Bus Selector1/1  "att_reset"
  gyro_B_correction/1 -> Signal Conversion2/1
  Signal Conversion4/1 -> Bus Creator/1  "att_reset"
  Constant/1 -> Signal Conversion1/1
  Bus Selector/1 -> Terminator2/1  "<gyro_B_rad/s_LPF>"

== system main_RI_LIEKF/State estimation/distribute CF/distribute CF/Correct ==
  Sensor_Data : Inport
  Rotation_Data : Inport  Port=2
  Attitude_Correction : Subsystem
  Subsystem2 : Subsystem
  att_B_correction : Outport
  bias_g_B_correction : Outport  Port=2
  wires:
  Attitude_Correction/1(att_B_correction) -> att_B_correction/1, Subsystem2/2(att_B_correction)
  Sensor_Data/1 -> Subsystem2/1(Sensor_Data), Attitude_Correction/1(Sensor_Data)
  Subsystem2/1(bias_g_B_correction) -> bias_g_B_correction/1
  Rotation_Data/1 -> Attitude_Correction/2(Rotation_Data)

== system main_RI_LIEKF/State estimation/distribute CF/distribute CF/Translation_estimate ==
  RotationData : Inport
  Sensor_data : Inport  Port=2
  Add : Sum  Inputs=++-
  Bus Creator2 : BusCreator  Inputs=6
  Bus Selector : BusSelector  OutputSignals=TOF_Data.H_TOF_TD,GPS_Data.pos_D_gps,QGC_sensor_reinit,GPS_Data.fixtype_gps
  Bus Selector1 : BusSelector  OutputSignals=M_OB
  Compare To Constant : simulink/Logic and Bit Operations/Compare To Constant  relop=>=  const=1  OutDataTypeStr=boolean
  Constant2 : Constant  Value=g0  OutDataTypeStr=single
  Demux : Demux  Outputs=2
  Demux1 : Demux  Outputs=2
  Demux2 : Demux  Outputs=3
  Detect Increase : simulink/Logic and Bit Operations/Detect Increase  vinit=0.0  OutDataTypeStr=boolean
  Gain : Gain  Gain=-1
  KalmanFilter_altitude : ctrlSharedLib/Kalman Filter  TimeDomain=Discrete-Time  UseCurrentEstimator=on  ModelSource=Individual A, B, C, D matrices  ModelSourceVariable=sys  A=[1 0.01 0; 0 1 -0.01;0 0 1-1/50;]  B=[0;0.01;0]  C=[1 0 0]  D=[0]  NumberOfStates=2  NumberOfInputs=2  NumberOfOutputs=2  InitialEstimateSource=Dialog  X0=[0 0 0]  P0=10  UseK=off  UseGH=on  NumberOfProcessNoiseInputs=2  G=diag([0;1;1])  TimeInvariantG=on  H=0  TimeInvariantH=on  Q=diag([0;5e-3;5e-4])  TimeInvariantQ=on  R=10  TimeInvariantR=on  N=0  TimeInvariantN=on  AddInputPort=on  AddEnablePort=on  ExternalReset=Rising  OutputEstimatedY=off  OutputP=off  Ts=-1
  Memory : Memory
  Rxy_Horizontal_estimation : Subsystem
  Scope : Scope  NumInputPorts=2
  Sensor_data1 : InportShadow  Port=2
  V_Horizontal_estimation : Subsystem
  Zero-Order Hold{,1..3} (4 alike) : ZeroOrderHold  SampleTime=0.01
  translate to N : Subsystem
  TranslationData : Outport
  wires:
  RotationData/1 -> Bus Selector1/1, translate to N/1(RotationData)
  Bus Creator2/1 -> TranslationData/1
  Demux1/2 -> Bus Creator2/5  "pe_m"
  Demux1/1 -> Bus Creator2/4  "pn_m"
  Demux/2 -> Bus Creator2/2  "ve_m/s"
  Demux/1 -> Bus Creator2/1  "vn_m/s"
  translate to N/2(accel_Vertical_predict) -> [accel_Vertical_predict]
  V_Horizontal_estimation/3(GPS_v_enable) -> Rxy_Horizontal_estimation/2(Enable)
  V_Horizontal_estimation/2(V_n&e) -> Rxy_Horizontal_estimation/1(Vn)
  V_Horizontal_estimation/1(vxy_estimout) -> Demux/1  "v_ne_"
  translate to N/1(accel_Horizontal_predict) -> V_Horizontal_estimation/1(An)
  Rxy_Horizontal_estimation/1(R_n&e) -> Demux1/1
  Sensor_data/1 -> translate to N/2(Sensor_data), V_Horizontal_estimation/2(Sensor_data2), Rxy_Horizontal_estimation/3(Sensor_data2)
  Sensor_data1/1 -> Bus Selector/1
  KalmanFilter_altitude/1 -> Demux2/1
  Demux2/1 -> Gain/1
  Zero-Order Hold/1 -> KalmanFilter_altitude/1
  Zero-Order Hold1/1 -> KalmanFilter_altitude/2
  Demux2/2 -> Bus Creator2/3  "vd_m/s"
  Gain/1 -> Bus Creator2/6  "H_m"
  [accel_Vertical_predict] -> Scope/1, Add/1
  Add/1 -> Zero-Order Hold/1
  Demux2/3 -> Memory/1
  Memory/1 -> Add/3, Scope/2
  Constant2/1 -> Add/2
  Bus Selector/3 -> Detect Increase/1  "<QGC_sensor_reinit>"
  Detect Increase/1 -> Zero-Order Hold3/1
  Bus Selector/4 -> Zero-Order Hold2/1  "<fixtype_gps>"
  Compare To Constant/1 -> KalmanFilter_altitude/3
  Zero-Order Hold2/1 -> Compare To Constant/1
  Bus Selector/2 -> Zero-Order Hold1/1  "<pos_D_gps>"
  Zero-Order Hold3/1 -> KalmanFilter_altitude/4
  Bus Selector1/1 -> Rxy_Horizontal_estimation/4(Cbn)  "<M_OB>"

== system main_RI_LIEKF/State estimation/distribute CF/distribute CF/Update ==
  note: 比例环节
  att_B_correction : Inport
  bias_g_correction : Inport  Port=2
  RF_Data : Inport  Port=3
  Sensor_Data : Inport  Port=4
  Attitude_Update : Subsystem
  Bus Selector : BusSelector  OutputSignals=IMU_Data.gyro_B_rad/s_LPF
  Bus Selector1 : BusSelector  OutputSignals=att_reset,quat_0
  Gain : Gain
  Gyro_Bias_Update : Subsystem
  Saturation : Saturate  UpperLimit=0.1  LowerLimit=-0.1
  Scope : Scope
  Scope1 : Scope
  Sum2 : Sum  Inputs=|++
  att_quat : Outport
  DCM_OB : Outport  Port=2
  bias_g : Outport  Port=3
  gyro_B_correction : Outport  Port=4
  wires:
  Sensor_Data/1 -> Bus Selector/1
  Sum2/1 -> Attitude_Update/3(att_B_correction)
  Bus Selector/1 -> Gyro_Bias_Update/2(gyr_B_radPs)  "<gyro_B_rad/s_LPF>"
  bias_g_correction/1 -> Gyro_Bias_Update/1(bias_g_correction)
  Attitude_Update/1(att_quat) -> att_quat/1
  Attitude_Update/2(DCM_OB) -> DCM_OB/1
  Gyro_Bias_Update/2(bias_g) -> Scope/1, bias_g/1
  RF_Data/1 -> Bus Selector1/1  "att_reset"
  Bus Selector1/1 -> Attitude_Update/1(att_reset)  "<att_reset>"
  Bus Selector1/2 -> Attitude_Update/2(quat_0)  "<quat_0>"
  Gyro_Bias_Update/1(gyr_B_correction) -> gyro_B_correction/1, Sum2/2
  att_B_correction/1 -> Gain/1
  Gain/1 -> Saturation/1, Scope1/1
  Saturation/1 -> Sum2/1

== system main_RI_LIEKF/State estimation/distribute CF/distribute CF/初始化 ==
  Sensor_Data : Inport
  Attitude_Reset : Subsystem
  Bus Creator : BusCreator  Inputs=2
  Scope : Scope
  Scope1 : Scope
  Subsystem : Subsystem
  RF_data : Outport
  wires:
  Attitude_Reset/1(att_reset) -> Subsystem/Enable, Bus Creator/1, Scope/1  "att_reset"
  Bus Creator/1 -> RF_data/1
  Subsystem/1(quat_0) -> Scope1/1, Bus Creator/2  "quat_0"
  Sensor_Data/1 -> Subsystem/1(sensor_data), Attitude_Reset/1(Sensor_Data)

== system main_RI_LIEKF/Sensor_Data_Process/Magn_Data_Process1/Mag_Data_Process/Mag_Quality_Estimate/Mag_Quality ==
  nominal_inc_deg : Inport
  mag_normalized_O : Inport  Port=2
  Inclination_Quality_Estimate : Subsystem
  Intensity_Quality_Estimate : Subsystem
  MinMax : MinMax  Inputs=2
  低通滤波 : Subsystem  mask{fc=5, zeta=0.707}
      mask prompts: fc "Cut-off frequence"; zeta "Damping factor"
      mask DialogControl ParameterGroupVar Prompt: 参数
  mag_quality : Outport  PortDimensions=1  VectorParamsAs1DForOutWhenUnconnected=off
  wires:
  Intensity_Quality_Estimate/1(intensity_quality) -> MinMax/2  "mag_int_quality"
  nominal_inc_deg/1 -> Inclination_Quality_Estimate/1(nominal_inc_deg)
  Inclination_Quality_Estimate/1(inclination_quality) -> MinMax/1  "mag_inc_quality"
  mag_normalized_O/1 -> Inclination_Quality_Estimate/2(mag_normalized_O), Intensity_Quality_Estimate/1(mag_normalized_O)
  MinMax/1 -> 低通滤波/1(u)
  低通滤波/1(y) -> mag_quality/1

== system main_RI_LIEKF/Sensor_Data_Process/Magn_Data_Process1/Mag_Data_Process/WMM_Compensation/Normlize ==
  In1 : Inport
  Constant : Constant  OutDataTypeStr=Inherit: Inherit via back propagation
  Data Type Duplicate : DataTypeDuplicate
  Demux : Demux  Outputs=[-1 1]
  Divide : Product  Inputs=*/
  Ground : Ground
  Math Function : Math  Operator=square  SignedPower=on  OutDataTypeStr=Inherit: Inherit via internal rule
  Math Function1 : Math  Operator=sqrt  SignedPower=on
  Mux : Mux  Inputs=2
  Mux1 : Mux  Inputs=2
  Product : Product  RndMeth=Zero  OutDataTypeStr=Inherit: Same as first input
  Sum of Elements : Sum  Inputs=+
  Switch : Switch  Criteria=u2 > Threshold  SaturateOnIntegerOverflow=off  InputSameDT=off
  Out1 : Outport  PortDimensions=3
  wires:
  Mux/1 -> Switch/1
  Ground/1 -> Product/2
  In1/1 -> Mux/1, Math Function/1, Product/1, Data Type Duplicate/2
  Sum of Elements/1 -> Math Function1/1
  Product/1 -> Mux1/1
  Math Function1/1 -> Switch/2, Mux/2
  Demux/2 -> Divide/2
  Switch/1 -> Demux/1
  Mux1/1 -> Switch/3
  Math Function/1 -> Sum of Elements/1
  Constant/1 -> Mux1/2, Data Type Duplicate/1
  Demux/1 -> Divide/1
  Divide/1 -> Out1/1

== system main_RI_LIEKF/Sensor_Data_Process/Magn_Data_Process1/Mag_Data_Process/WMM_Compensation/psi2DCMz ==
  In1 : Inport
  Constant : Constant  OutDataTypeStr=Inherit: Inherit via back propagation
  Constant{1..4} (4 alike) : Constant  Value=0  OutDataTypeStr=Inherit: Inherit via back propagation
  Gain1 : Gain  Gain=-1
  Trigonometric Function : Trigonometry
  Trigonometric Function1 : Trigonometry  Operator=cos
  Trigonometric Function2 : Trigonometry
  Trigonometric Function3 : Trigonometry  Operator=cos
  Vector Concatenate : Concatenate  NumInputs=3  Mode=Multidimensional array  ConcatenateDimension=2
  Vector Concatenate1 : Concatenate  NumInputs=3  Mode=Multidimensional array
  Vector Concatenate2 : Concatenate  NumInputs=3  Mode=Multidimensional array
  Vector Concatenate3 : Concatenate  NumInputs=3  Mode=Multidimensional array
  Out1 : Outport
  wires:
  Constant1/1 -> Vector Concatenate3/2
  Constant/1 -> Vector Concatenate3/3
  Vector Concatenate/1 -> Out1/1
  Trigonometric Function2/1 -> Gain1/1
  Constant2/1 -> Vector Concatenate3/1
  In1/1 -> Trigonometric Function3/1, Trigonometric Function2/1, Trigonometric Function/1, Trigonometric Function1/1
  Trigonometric Function/1 -> Vector Concatenate1/2
  Vector Concatenate2/1 -> Vector Concatenate/2
  Vector Concatenate1/1 -> Vector Concatenate/1
  Vector Concatenate3/1 -> Vector Concatenate/3
  Gain1/1 -> Vector Concatenate2/1
  Constant3/1 -> Vector Concatenate1/3
  Trigonometric Function1/1 -> Vector Concatenate1/1
  Constant4/1 -> Vector Concatenate2/3
  Trigonometric Function3/1 -> Vector Concatenate2/2

== system main_RI_LIEKF/Sensor_Data_Process/Magn_Data_Process1/Mag_Data_Process/WMM_Compensation/safe_divide ==
  u1 : Inport
  u2 : Inport  Port=2
  Constant1 : Constant  VectorParams1D=off  OutDataTypeStr=single
  Divide1 : Product  Inputs=*/
  MinMax : MinMax  Function=max  Inputs=2
  y : Outport  VectorParamsAs1DForOutWhenUnconnected=off
  wires:
  MinMax/1 -> Divide1/2
  Constant1/1 -> MinMax/1
  Divide1/1 -> y/1
  u2/1 -> MinMax/2
  u1/1 -> Divide1/1

== system main_RI_LIEKF/State estimation/0609bk/Error State Kalman Filter/Extended Kalman Filter1/Correct1 ==
  yMeas : Inport  SampleTime=SampleTime
  R : Inport  Port=2  SampleTime=SampleTime
  uMeas : Inport  Port=3  SampleTime=SampleTime
  uBlockOrdering : Inport  Port=4  SampleTime=SampleTime
  Enable : EnablePort
  Correct : MATLAB Function  TreatAsAtomicUnit=on
  Data Store ReadP : DataStoreRead  DataStoreName=P  IndexOptions=Index vector (dialog)  Indices=1  OutputSizes=1
  Data Store ReadX : DataStoreRead  DataStoreName=x  IndexOptions=Index vector (dialog)  Indices=1  OutputSizes=1
  Data Store WriteP : DataStoreWrite  DataStoreName=P  IndexOptions=Index vector (dialog)  Indices=1  OutputSizes=1
  Data Store WriteX : DataStoreWrite  DataStoreName=x  IndexOptions=Index vector (dialog)  Indices=1  OutputSizes=1
  IGG_check : Subsystem  Commented=on
  R1 : InportShadow  Port=2  SampleTime=SampleTime
  RegisterSimulinkFcn : S-Function  FunctionName=ekfukfRegisterSimulinkFcn  Parameters=int32(3), 1, pM.HasAdditiveNoise, SampleTime, DataType, SLFcnsToRegister  SFunctionDeploymentMode=off  EnableBusSupport=off
  Scope1 : Scope
  yMeas1 : InportShadow  SampleTime=SampleTime
  yBlockOrdering : Outport  VectorParamsAs1DForOutWhenUnconnected=off
  wires:
  uMeas/1 -> Correct/5(uMeas)
  uBlockOrdering/1 -> Correct/6("blockOrdering ")
  Correct/3(blockOrdering) -> yBlockOrdering/1
  Correct/1(xNew) -> Data Store WriteX/1
  R/1 -> RegisterSimulinkFcn/3, Correct/4(R)
  yMeas/1 -> RegisterSimulinkFcn/2, Correct/3(yMeas)
  Correct/2(P) -> Data Store WriteP/1
  Data Store ReadP/1 -> IGG_check/1(Pk/k_1), Correct/2("P ")
  Data Store ReadX/1 -> IGG_check/3(X), Correct/1(x), RegisterSimulinkFcn/1
  yMeas1/1 -> IGG_check/2(yMeas)
  R1/1 -> IGG_check/4(R)
  IGG_check/2(w) -> Scope1/1

== system main_RI_LIEKF/State estimation/0609bk/Error State Kalman Filter/Extended Kalman Filter1/Output ==
  uBlockOrdering : Inport
  Data Store Read : DataStoreRead  DataStoreName=x  IndexOptions=Index vector (dialog)  Indices=1  OutputSizes=1
  Data Store Read1 : DataStoreRead  DataStoreName=P  IndexOptions=Index vector (dialog)  Indices=1  OutputSizes=1
  MATLAB Function : MATLAB Function  TreatAsAtomicUnit=on
  x : Outport  VectorParamsAs1DForOutWhenUnconnected=off
  P : Outport  Port=2  VectorParamsAs1DForOutWhenUnconnected=off
  yBlockOrdering : Outport  Port=3  VectorParamsAs1DForOutWhenUnconnected=off
  wires:
  MATLAB Function/1(P) -> P/1
  uBlockOrdering/1 -> yBlockOrdering/1
  Data Store Read1/1 -> MATLAB Function/1(S)
  Data Store Read/1 -> x/1
